simulink model "MultiVehicleModel"  (R2014a)
settings: Solver=ode1  StartTime=0.0  StopTime=inf  FixedStep=simPars.SampleTime  RelTol=1e-3
undefined symbols (not defined in the file or in its folder): DiscIntNeverNeededParam, Earth, Env, eul_0, FWFleet, GVFleet, m, RCFleet, s, WGS84
undefined symbols (not defined in the file): simPars
libraries: simulink x26, aerolibtransform2 x7, instrumentlib x6, Actuator_Lib x5, aerolib6dofsys x4, etargetslib x3, aerolibasang x3, aerolibconvert2 x2, aerolibutil x1, aerolibatmos2 x1, aerolibobsolete x1, aerolibgravity2 x1
(part 4 of 4)

== matlab function MultiVehicleModel/Rotorcraft fleet/Multiple Rotorcraft/Guidance /flight manager - ARDRone outer loop ==
  data: psiRef output; hRef output; waypoint1 input; waypoint2 input; psi input; Pned input; h input; fcn input; XeRef output; YeRef output; time input; IC output; newMissionFlag output
function [psiRef, hRef,  XeRef, YeRef, IC, newMissionFlag]       = fcn(waypoint1, waypoint2, psi, Pned, h, fcn, time )
%#codegen

nPoints = size(waypoint1, 2) ;
waypoint = [waypoint1 ;waypoint2] ; 

waypoint(3,:) = -waypoint(3,:) ; 
IC = waypoint(1:4,1) ; 
% persitent variable used to keep trak of next waypoint
persistent wpointer;

% persitent variable used to keep track of operation mode.
% mode = 1: tracking next waypoint
% mode = 2: tracking an intermediate waypoint to guarantee
persistent mode;

% auxilary waypoint coordinates for operation in mode 2
persistent wpointAux;


% time zero at each target
persistent t0 ;

if isempty(wpointer)
    wpointer = 1;
end

if isempty(mode)
    mode = 1;
end

if isempty(wpointAux)
    wpointAux = zeros(2, 2);
end

if isempty(t0)
    t0 = 0;
end

newMissionFlag = 0;
switch  fcn
    case 1
        wpointer  = 1;
        newMissionFlag = 1;
        disp('resetting mission ... ')
    otherwise
end


% a waypoint is reached if the distance to the aircraft is less than 10 m
if (mode ==1 && norm(Pned(1:2) - waypoint(1:2, wpointer) )< 0.1 && ...
        norm(h - waypoint(3, wpointer)) < 0.1  && norm(psi - waypoint(4, wpointer) )< 5*pi/180   )
    
    if(wpointer ~= nPoints)
        
        if (t0 ==0)
            t0 = time;
        else
            if (time - t0 > waypoint(5, wpointer))
                
                 if(wpointer < nPoints)
                    wpointer = wpointer+ 1;
                    t0 = 0;
                 end
                
            end
        end
        
        
        
    end
    
       
    
end

hRef = waypoint(3, wpointer) ;
psiRef = waypoint(4, wpointer) ;
XeRef = waypoint(1, wpointer) ;
YeRef = waypoint(2, wpointer) ;

== matlab function MultiVehicleModel/Mission planning and monitoring - Network/Mission Plan Generation for ground vehicle fleet Runs on the server // cloud/Fleet Waypoint Reading from UDP/data processing  ==
  data: uavID input; functionID input; dataUAV input; dataFleet output; fcnFleet output; status input; nAC parameter double size=[1,1]; LLA0 input
function [dataFleet,fcnFleet] = fcn(uavID, functionID , dataUAV, status, nAC, LLA0)
%#codegen

nWPs = 100; 
fcnFleet = zeros(nAC,1) ;

persistent waypointsFleet; 

if isempty(waypointsFleet)
    waypointsFleet = zeros(3,nWPs, nAC);  
    waypointsFleet(1,:,:) = ones(1,nWPs, nAC)*LLA0(1) ; 
    waypointsFleet(2,:,:) = ones(1,nWPs, nAC)*LLA0(2) ; 
    waypointsFleet(3,:,:) = ones(1,nWPs, nAC)*LLA0(3) ; 
end

switch functionID
    case 1 % setting waypoint list of a UAV into database
        if (uavID <= nAC )
            waypointsFleet(:,1:nWPs,uavID) = reshape(dataUAV, 3 ,nWPs  ); 
            if status ==1
                fcnFleet(uavID) =functionID ; % reset
                disp('status GV = 1') ;
            end
        end
        
        
    otherwise
        
        
    
end


dataFleet = waypointsFleet(1:3,:,:);

== matlab function MultiVehicleModel/Ground Vehicle fleet/Model of ground vehicle fleet/Very simple car model/MATLAB Function ==
  data: u input; xNorthDot output; psi input; yEastDot output
function [xNorthDot, yEastDot ] = fcn(u, psi)
%#codegen

xNorthDot = u*cos(psi);
yEastDot = u*sin(psi);

== matlab function MultiVehicleModel/Ground Vehicle fleet/Model of ground vehicle fleet/Guidance algorithm/Ground track angle computation based on waypoints ==
  data: vCmd output; waypoint input; Pned input; psiTarget output; fcn input
function [vCmd ,psiTarget]     = fcn(waypoint, Pned, fcn )
%#codegen

nPoints = size(waypoint, 2) ;

%size(waypoint)
% persitent variable used to keep trak of next waypoint
persistent wpointer; 

persistent psiRec; 

% auxilary waypoint coordinates for operation in mode 2
persistent wpointAux; 

if isempty(wpointer) 
wpointer = 1

end

if isempty(psiRec) 
psiRec = atan2( waypoint(2,wpointer) - Pned(2) , waypoint(1,wpointer) - Pned(1)) ;
end


switch  fcn
    case 1
        wpointer  = 1;
        disp('resetting mission GV ... ')
        psiRec = atan2( waypoint(2,wpointer) - Pned(2) , waypoint(1,wpointer) - Pned(1)) ;
    otherwise
end

vCmd = 18;

% a waypoint is reached if the distance to the aircraft is less than 1 m
if ( norm(Pned(1:2) - waypoint(1:2, wpointer) )< 1 && (wpointer < nPoints) ) 
    
       wpointer = wpointer + 1 ;
       vCmd = 0;
       psiRec = atan2( waypoint(2,wpointer) - Pned(2) , waypoint(1,wpointer) - Pned(1)) ;
end

psiTarget = psiRec; 

% psiTarget from 0 to 360 deg only
%{
if (psiTarget <0)
    psiTarget = 2*pi+psiTarget ; 
end
%}

if (waypoint(3,wpointer) >0  || wpointer>=nPoints )
    vCmd = 0; 
   
end

%{
psiTarget
vCmd
Pned
waypoint(1:2, wpointer)
wpointer
%}

== matlab function MultiVehicleModel/Rotorcraft fleet/Multiple Rotorcraft/ARDrone model1/Velocity from vehicle body frame to inertial NED  frame ==
  data: Vx input; Vy input; Vel_xy output; psi input
function Vel_xy = fcn(Vx, Vy , psi)
%#codegen
Vel_b= [Vx;Vy] ; 
T = [cos(psi) -sin(psi) ; sin(psi) cos(psi)] ; 
Vel_xy = T*Vel_b;

== matlab function MultiVehicleModel/Rotorcraft fleet/Multiple Rotorcraft/vehicle controller1/normalize angle between -180 and 180 deg ==
  data: angleIn input; angleOut output
function angleOut = fcn(angleIn)
%#codegen

angleOut = mod(angleIn, 2*pi) ;
if angleOut > 180
    angleOut = 2*pi - angleOut ; 
end
